simulink model "sds1104receiver"  (R2023a)
settings: Solver=VariableStepAuto  StartTime=0.0  StopTime=inf  RelTol=1e-3
settings Model: Creator=User  LastModifiedBy=User

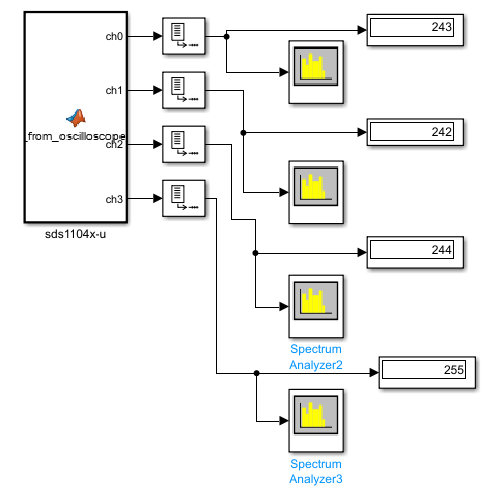
[thumbnail: Simulink's stored preview of the top-level diagram]
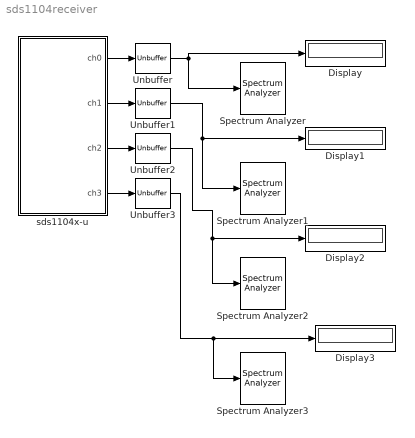
== system sds1104receiver ==
  Display{,1..3} (4 alike) : Display
  Spectrum Analyzer : SpectrumAnalyzer  WindowPosition=[1692.000000,114.000000,800.000000,500.000000,]  Visible=on  ScopeFrameLocation=window  SampleRateSource=Property  SampleRate=44.1e3  PlotAsTwoSidedSpectrum=off  FrequencySpan=Start and stop frequencies  StartFrequency=20  StopFrequency=20e3  YLimits=[-14.60311564,88.0301966]  ColorLimits=[-20 80]  DefaultConfigurationName=spbscopes.SpectrumAnalyzerBlockCfg  IsFrequencyInputMode=0  FrequencyVectorPort=0  FrequencyVectorFromPort=0  FrequencyInputRBWPort=0  FrequencyInputRBWFromPort=0
  Spectrum Analyzer1 : SpectrumAnalyzer  WindowPosition=[1692.000000,114.000000,800.000000,500.000000,]  ScopeFrameLocation=window  SampleRateSource=Property  SampleRate=44.1e3  PlotAsTwoSidedSpectrum=off  FrequencySpan=Start and stop frequencies  StartFrequency=20  StopFrequency=20e3  YLimits=[-14.60311564,88.0301966]  ColorLimits=[-20 80]  DefaultConfigurationName=spbscopes.SpectrumAnalyzerBlockCfg  IsFrequencyInputMode=0  FrequencyVectorPort=0  FrequencyVectorFromPort=0  FrequencyInputRBWPort=0  FrequencyInputRBWFromPort=0
  Spectrum Analyzer2 : SpectrumAnalyzer  WindowPosition=[1692.000000,114.000000,800.000000,500.000000,]  ScopeFrameLocation=window  SampleRateSource=Property  SampleRate=44.1e3  PlotAsTwoSidedSpectrum=off  FrequencySpan=Start and stop frequencies  StartFrequency=20  StopFrequency=20e3  YLimits=[-14.60311564,88.0301966]  ColorLimits=[-20 80]  DefaultConfigurationName=spbscopes.SpectrumAnalyzerBlockCfg  IsFrequencyInputMode=0  FrequencyVectorPort=0  FrequencyVectorFromPort=0  FrequencyInputRBWPort=0  FrequencyInputRBWFromPort=0
  Spectrum Analyzer3 : SpectrumAnalyzer  WindowPosition=[1692.000000,114.000000,800.000000,500.000000,]  ScopeFrameLocation=window  SampleRateSource=Property  SampleRate=44.1e3  PlotAsTwoSidedSpectrum=off  FrequencySpan=Start and stop frequencies  StartFrequency=20  StopFrequency=20e3  YLimits=[-14.60311564,88.0301966]  ColorLimits=[-20 80]  DefaultConfigurationName=spbscopes.SpectrumAnalyzerBlockCfg  IsFrequencyInputMode=0  FrequencyVectorPort=0  FrequencyVectorFromPort=0  FrequencyInputRBWPort=0  FrequencyInputRBWFromPort=0
  Unbuffer{,1..3} (4 alike) : Unbuffer
  sds1104x-u : MATLAB Function  TreatAsAtomicUnit=on  SystemSampleTime=8192/500000
  wires:
  sds1104x-u/1(ch0) -> Unbuffer/1
  sds1104x-u/2(ch1) -> Unbuffer1/1
  sds1104x-u/3(ch2) -> Unbuffer2/1
  sds1104x-u/4(ch3) -> Unbuffer3/1
  Unbuffer/1 -> Display/1, Spectrum Analyzer/1
  Unbuffer1/1 -> Spectrum Analyzer1/1, Display1/1
  Unbuffer2/1 -> Spectrum Analyzer2/1, Display2/1
  Unbuffer3/1 -> Spectrum Analyzer3/1, Display3/1

== matlab function sds1104receiver/sds1104x-u ==
  data: ch0 output; ch1 output; ch2 output; ch3 output
% this is for simulink matlab module
function [ch0,ch1,ch2,ch3] = read_file_from_oscilloscope_receiver()
    persistent buf
    N = 7000000;
    if isempty(buf)
        buf = zeros(4*N,1,'uint8');
    end
    % Call helper function to get latest data
    buf = read_file_helper(N);
    ch0 = buf(1:N);
    ch1 = buf(N+1:2*N);
    ch2 = buf(2*N+1:3*N);
    ch3 = buf(3*N+1:4*N);
end
